simulink model "Control_DC_Motor"  (R2022b)
settings: Solver=ode1  StartTime=0.0  StopTime=10  FixedStep=0.001  RelTol=1e-3
InitFcn:
  | R = 1;
  | L = 0.5;
  | K = 0.01;
  | b = 0.1;
  | J = 0.01;
  | Kt = 0.01;
  | 
  | A = [-R/L -K/L; Kt/J -b/J];
  | B = [1/L; 0];
  | C = [0 1];
  | D = 0;
  | 
  | [Num Den] = ss2tf(A,B,C,D);
  | G = tf(Num, Den);
libraries: slpidlib x1
settings Model: Creator=user  LastModifiedBy=user

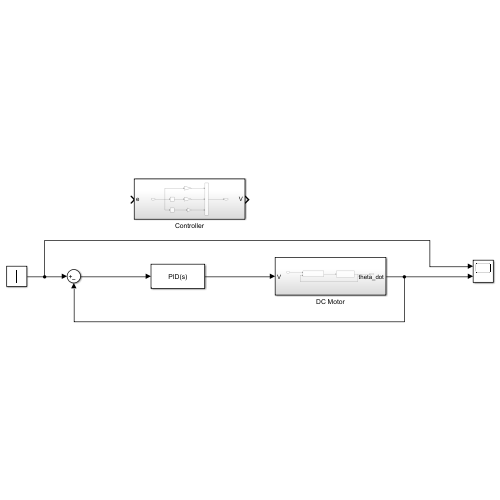
[thumbnail: Simulink's stored preview of the top-level diagram]
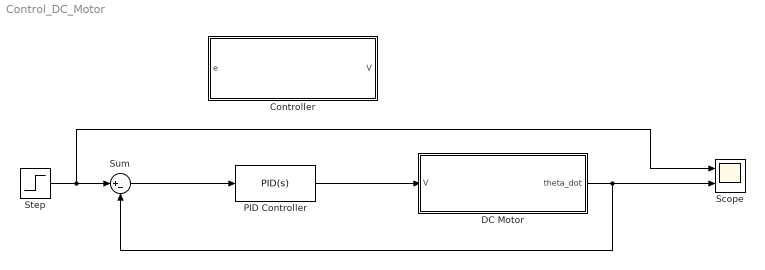
== system Control_DC_Motor ==
  Controller : Subsystem
  DC Motor : Subsystem
  PID Controller : slpidlib/PID Controller  Controller=PID  Form=Parallel  TimeDomain=Continuous-time  UseExternalTs=off  SampleTime=-1  IntegratorMethod=Forward Euler  FilterMethod=Forward Euler  ControllerParametersSource=internal  P=4.18547301272689  I=12.0378710949144  UseKiTs=off  D=0  N=100  UseFilter=on  TunerSelectOption=Transfer Function Based (PID Tuner App)  InitialConditionSource=internal  InitialConditionForIntegrator=0  InitialConditionForFilter=0  DifferentiatorICPrevScaledInput=0  ExternalReset=none  TrackingMode=off  Kt=1  LimitOutput=off  SatLimitsSource=internal  UpperSaturationLimit=inf  LowerSaturationLimit=-inf  LinearizeAsGain=on  AntiWindupMode=none  Kb=1  LimitIntegrator=off  UpperIntegratorSaturationLimit=inf  LowerIntegratorSaturationLimit=-inf  POutMin=[]  POutMax=[]  IOutMin=[]  IOutMax=[]  DOutMin=[]  DOutMax=[]  NOutMin=[]  NOutMax=[]  SumOutMin=[]  SumOutMax=[]  SaturationOutMin=[]  SaturationOutMax=[]  PParamMin=[]  PParamMax=[]  IParamMin=[]  IParamMax=[]  DParamMin=[]  DParamMax=[]  NParamMin=[]  NParamMax=[]  KbParamMin=[]  KbParamMax=[]  KtParamMin=[]  KtParamMax=[]  KbOutMin=[]  KbOutMax=[]  KtOutMin=[]  KtOutMax=[]  IntegratorOutMin=[]  IntegratorOutMax=[]  FilterOutMin=[]  FilterOutMax=[]  SumI1OutMin=[]  SumI1OutMax=[]  SumI2OutMin=[]  SumI2OutMax=[]  SumI3OutMin=[]  SumI3OutMax=[]  SumI4OutMin=[]  SumI4OutMax=[]  SumDOutMin=[]  SumDOutMax=[]  DifferentiatorOutMin=[]  DifferentiatorOutMax=[]  FilterDiffOutCoefMin=[]  FilterDiffOutCoefMax=[]  ReciprocalOutMin=[]  ReciprocalOutMax=[]  SumDenOutMin=[]  SumDenOutMax=[]  SumNumOutMin=[]  SumNumOutMax=[]  DivideOutMin=[]  DivideOutMax=[]  UdiffTsProdOutMin=[]  UdiffTsProdOutMax=[]  NTsProdOutMin=[]  NTsProdOutMax=[]  UintegralTsProdOutMin=[]  UintegralTsProdOutMax=[]  UngainTsProdOutMin=[]  UngainTsProdOutMax=[]  ClampingZeroOutDataTypeStr=Inherit: Inherit via back propagation  ClampingZeroOutMin=[]  ClampingZeroOutMax=[]  FilterDenConstantOutDataTypeStr=Inherit: Inherit via back propagation  FilterDenConstantOutMin=[]  FilterDenConstantOutMax=[]  PCopyOutDataTypeStr=Inherit: Inherit via back propagation  PCopyOutMin=[]  PCopyOutMax=[]  NCopyOutDataTypeStr=Inherit: Inherit via back propagation  NCopyOutMin=[]  NCopyOutMax=[]  IntegratorContinuousStateAttributes=''  IntegratorStateMustResolveToSignalObject=off  IntegratorRTWStateStorageClass=Auto  FilterContinuousStateAttributes=''  FilterStateMustResolveToSignalObject=off  FilterRTWStateStorageClass=Auto  ParallelPVariant=InternalParameters  IdealPVariant=Disabled  IVariant=InternalParameters  DVariant=InternalParameters  IntegratorVariant=Continuous  SatVariant=Disabled  AWVariant=Passthrough  PCopyVariant=Disabled  TRVariant=Disabled  FdbkBlocksVariant=Forward  IdealPFdbkVariant=Disabled  SatFdbkVariant=Disabled  DerivativeFilterVariant=ContFilter  NVariant=InternalParameters  NCopyVariant=Disabled  FilterICVariant=InternalICsFilter  IntegratorICVariant=InternalICs  ExternalResetVariant=Disabled  TRSumVariant=Passthrough  SumFdbkVariant=Disabled  SumVariant=Sum_PID  TsampFilterVariant=InternalTs  TsampNgainVariant=Passthrough  TsampIntegralVariant=Passthrough  ExternalSaturationOutDataTypeStr=Inherit: Same as second input
  Scope : Scope  NumInputPorts=2
  Step : Step  After=10  SampleTime=0
  Sum : Sum  Inputs=|+-
  wires:
  Step/1 -> Scope/1, Sum/1
  DC Motor/1(theta_dot) -> Sum/2, Scope/2
  PID Controller/1 -> DC Motor/1(V)
  Sum/1 -> PID Controller/1

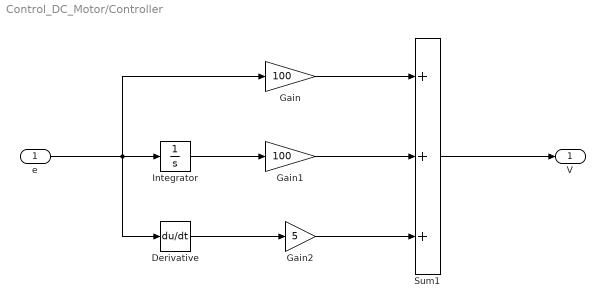
== system Control_DC_Motor/Controller ==
  e : Inport
  Derivative : Derivative
  Gain : Gain  Gain=100
  Gain1 : Gain  Gain=100
  Gain2 : Gain  Gain=5
  Integrator : Integrator
  Sum1 : Sum  Inputs=+++
  V : Outport
  wires:
  Gain1/1 -> Sum1/2
  Gain/1 -> Sum1/1
  e/1 -> Derivative/1, Integrator/1, Gain/1
  Sum1/1 -> V/1
  Derivative/1 -> Gain2/1
  Gain2/1 -> Sum1/3
  Integrator/1 -> Gain1/1

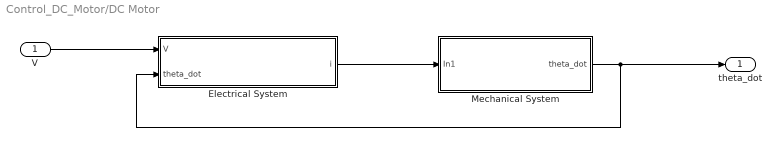
== system Control_DC_Motor/DC Motor ==
  V : Inport
  Electrical System : Subsystem
  Mechanical System : Subsystem
  theta_dot : Outport
  wires:
  Mechanical System/1(theta_dot) -> theta_dot/1, Electrical System/2(theta_dot)
  V/1 -> Electrical System/1(V)
  Electrical System/1(i) -> Mechanical System/1(In1)

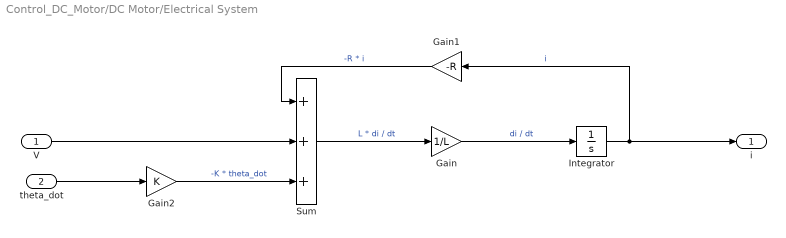
== system Control_DC_Motor/DC Motor/Electrical System ==
  V : Inport
  theta_dot : Inport  Port=2
  Gain : Gain  Gain=1/L
  Gain1 : Gain  Gain=-R
  Gain2 : Gain  Gain=K
  Integrator : Integrator
  Sum : Sum  Inputs=+++
  i : Outport
  wires:
  Gain1/1 -> Sum/1  "-R * i"
  Gain/1 -> Integrator/1  "di / dt"
  theta_dot/1 -> Gain2/1
  Gain2/1 -> Sum/3  "-K * theta_dot"
  Integrator/1 -> i/1, Gain1/1  "i"
  Sum/1 -> Gain/1  "L * di / dt"
  V/1 -> Sum/2

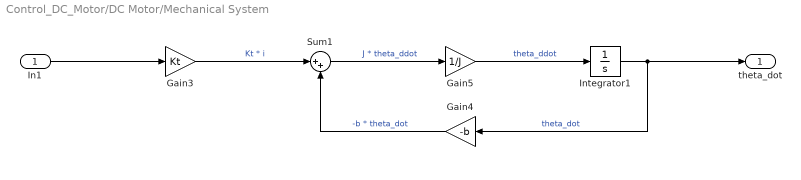
== system Control_DC_Motor/DC Motor/Mechanical System ==
  In1 : Inport
  Gain3 : Gain  Gain=Kt
  Gain4 : Gain  Gain=-b
  Gain5 : Gain  Gain=1/J
  Integrator1 : Integrator
  Sum1 : Sum  Inputs=|++
  theta_dot : Outport
  wires:
  In1/1 -> Gain3/1
  Gain5/1 -> Integrator1/1  "theta_ddot"
  Integrator1/1 -> theta_dot/1, Gain4/1  "theta_dot"
  Sum1/1 -> Gain5/1  "J * theta_ddot"
  Gain3/1 -> Sum1/1  "Kt * i"
  Gain4/1 -> Sum1/2  "-b * theta_dot"
